simulink model "lookup_test"  (R2017a)
settings: Solver=FixedStepDiscrete  StartTime=0.0  StopTime=1000  FixedStep=0.001  RelTol=1e-3
undefined symbols (not defined in the file or in its folder): DiscIntNeverNeededParam, F1, V1
libraries: eltreclib x1
settings Model: Creator=mayartmal  LastModifiedBy=mayartmal

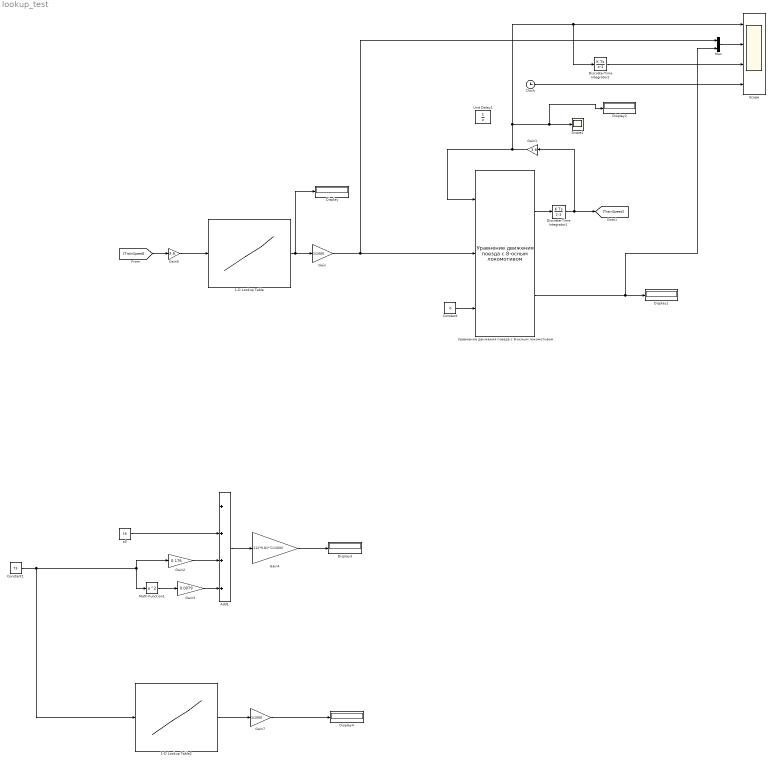
== system lookup_test ==
  1-D Lookup Table : Lookup_n-D  NumberOfTableDimensions=1  BreakpointsForDimension1=V1  Table=F1  InternalRulePriority=Speed  RndMeth=Simplest  InputSameDT=on
  1-D Lookup Table2 : Lookup_n-D  NumberOfTableDimensions=1  BreakpointsForDimension1=V1  Table=F1  InternalRulePriority=Speed  RndMeth=Simplest  InputSameDT=on
  Add1 : Sum  Inputs=++++
  Clock : Clock
  Constant : Constant  Value=0
  Constant1 : Constant  Value=73
  Discrete-Time Integrator1 : DiscreteIntegrator  InitialConditionSetting=State (most efficient)  SampleTime=-1  ICPrevOutput=DiscIntNeverNeededParam  ICPrevScaledInput=DiscIntNeverNeededParam
  Discrete-Time Integrator2 : DiscreteIntegrator  InitialConditionSetting=State (most efficient)  SampleTime=-1  ICPrevOutput=DiscIntNeverNeededParam  ICPrevScaledInput=DiscIntNeverNeededParam
  Display{,1..4} (5 alike) : Display
  Gain : Gain  Gain=1/1000
  Gain1 : Gain  Gain=3.6
  Gain2 : Gain  Gain=0.176
  Gain3 : Gain  Gain=0.0079
  Gain4 : Gain  Gain=112*9.81*(1/1000)
  Gain5 : Gain  Gain=3.6
  Gain7 : Gain  Gain=1/1000
  Math Function1 : Math  Operator=square  SaturateOnIntegerOverflow=on
  Mux : Mux  Inputs=2
  Scope : Scope  NumInputPorts=4
  Scope1 : Scope
  Unit Delay1 : UnitDelay  SampleTime=-1
  a0 : Constant  Value=16
  Уравнение движения поезда c 8-осным локомотивом : eltreclib/Уравнение движения поезда c 8-осным локомотивом  a0=16  a1=0.176  a2=0.0079  P=56*2
  wires:
  1-D Lookup Table/1 -> Display/1, Gain/1
  Constant1/1 -> 1-D Lookup Table2/1, Gain2/1, Math Function1/1
  Discrete-Time Integrator1/1 -> Gain1/1, [TrainSpeed]
  Уравнение движения поезда c 8-осным локомотивом/1 -> Discrete-Time Integrator1/1
  Constant/1 -> Уравнение движения поезда c 8-осным локомотивом/3
  Gain1/1 -> Discrete-Time Integrator2/1, Scope/1, Display2/1, Scope1/1, Уравнение движения поезда c 8-осным локомотивом/1
  Discrete-Time Integrator2/1 -> Scope/3
  Clock/1 -> Scope/4
  Gain/1 -> Mux/1, Уравнение движения поезда c 8-осным локомотивом/2
  Gain2/1 -> Add1/3
  Gain3/1 -> Add1/4
  Add1/1 -> Gain4/1
  a0/1 -> Add1/2
  ? -> Add1/1
  Math Function1/1 -> Gain3/1
  Gain4/1 -> Display3/1
  1-D Lookup Table2/1 -> Gain7/1
  Gain7/1 -> Display4/1
  Уравнение движения поезда c 8-осным локомотивом/2 -> Mux/2, Display1/1
  [TrainSpeed] -> Gain5/1
  Gain5/1 -> 1-D Lookup Table/1
  Mux/1 -> Scope/2
